simulink model "p4_state_space"  (R2025b)
settings: Solver=VariableStepAuto  StartTime=0.0  StopTime=5  RelTol=1e-3
values from neighbouring files (symbols this model uses):
  A = [-b/J, Kt/J ... (first row only)    [script_p1_to_p4.m]
  B = [0 ... (first row only)    [script_p1_to_p4.m]
  K_gain = place(A, B, DesiredPoles)    [script_p1_to_p4.m]
  Kr = -1 / (C * inv(A - B * K_gain) * B)    [script_p1_to_p4.m]
settings Model: Creator=Kittitouch Tantiwong  LastModifiedBy=Kittitouch Tantiwong

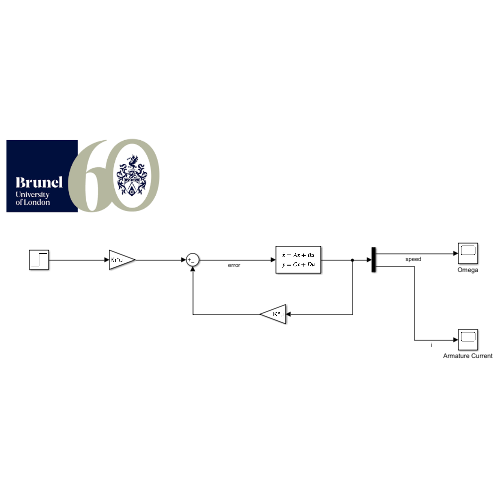
[thumbnail: Simulink's stored preview of the top-level diagram]
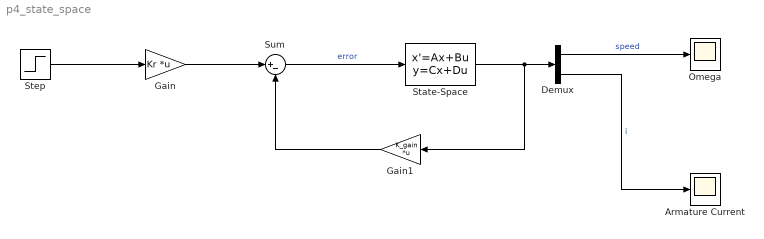
== system p4_state_space ==
  Armature Current : Scope
      settings: ActiveDisplayYMinimum=-1  ActiveDisplayYMaximum=1
  Demux : Demux  Outputs=2
  Gain : Gain  Gain=Kr  Multiplication=Matrix(K*u)
  Gain1 : Gain  Gain=K_gain  Multiplication=Matrix(K*u)
  Omega : Scope
      settings: ActiveDisplayYMinimum=-0.125  ActiveDisplayYMaximum=1.1250000000000002
  State-Space : StateSpace  A=A  B=B  C=[1 0; 0 1]  D=[0 ; 0]  InitialCondition=0  ParameterTunability=Unconstrained
  Step : Step  SampleTime=0
  Sum : Sum  Inputs=|+-
  wires:
  Step/1 -> Gain/1
  Sum/1 -> State-Space/1  "error"
  Gain/1 -> Sum/1
  State-Space/1 -> Gain1/1, Demux/1
  Demux/1 -> Omega/1  "speed"
  Gain1/1 -> Sum/2
  Demux/2 -> Armature Current/1  "i"
